simulink model "exp3"  (R2015a)
settings: Solver=ode45  StartTime=0.0  StopTime=10.0  RelTol=1e-3
settings Model: Creator=Rajib Kr paul  LastModifiedBy=Rajib Kr paul

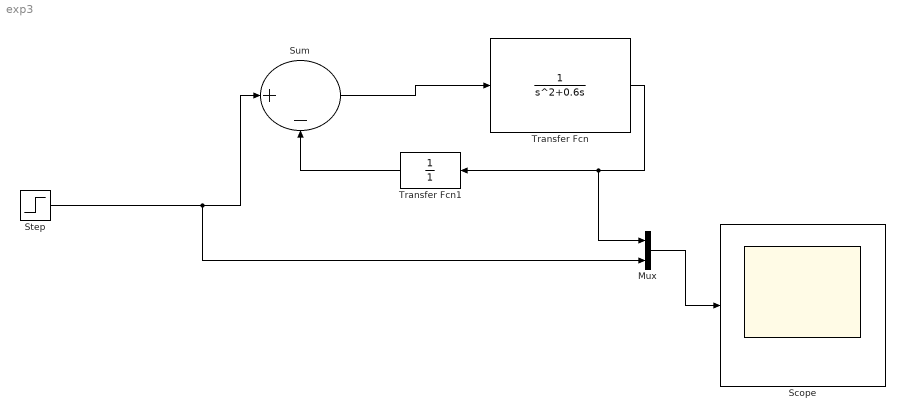
== system exp3 ==
  Mux : Mux  Inputs=2
  Scope : Scope
  Step : Step  Time=0  SampleTime=0
  Sum : Sum  Inputs=|+-
  Transfer Fcn : TransferFcn  Denominator=[1 0.6 0]
  Transfer Fcn1 : TransferFcn  Denominator=[1]
  wires:
  Step/1 -> Mux/2, Sum/1
  Sum/1 -> Transfer Fcn/1
  Transfer Fcn/1 -> Transfer Fcn1/1, Mux/1
  Mux/1 -> Scope/1
  Transfer Fcn1/1 -> Sum/2
